simulink model "LADRC2"  (R2023a)
settings: Solver=VariableStepAuto  StartTime=0.0  StopTime=10  RelTol=1e-3
settings Model: Creator=belov  LastModifiedBy=belov

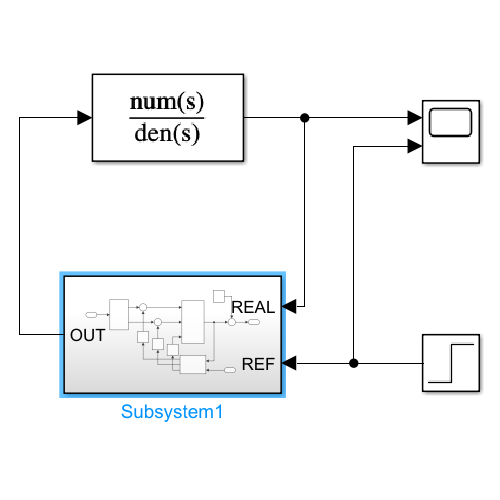
[thumbnail: Simulink's stored preview of the top-level diagram]
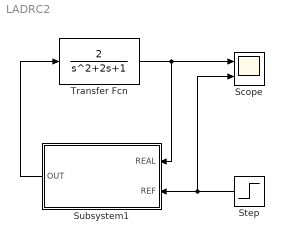
== system LADRC2 ==
  Scope : Scope  NumInputPorts=2
  Step : Step  SampleTime=0.001
  Subsystem1 : Subsystem
  Transfer Fcn : TransferFcn  Numerator=2
  wires:
  Step/1 -> Scope/2, Subsystem1/2(REF)
  Transfer Fcn/1 -> Subsystem1/1(REAL), Scope/1
  Subsystem1/1(OUT) -> Transfer Fcn/1

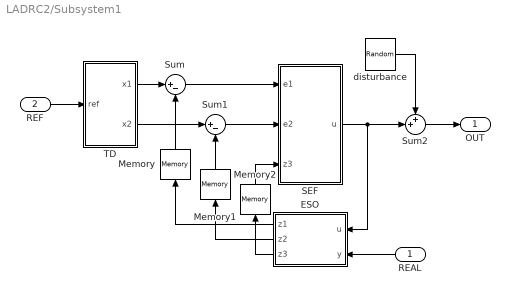
== system LADRC2/Subsystem1 ==
  REAL : Inport
  REF : Inport  Port=2  SampleTime=0.001
  ESO : MATLAB Function  TreatAsAtomicUnit=on  SystemSampleTime=0.001
  Memory : Memory
  Memory1 : Memory
  Memory2 : Memory
  SEF : MATLAB Function  TreatAsAtomicUnit=on  SystemSampleTime=0.001
  Sum : Sum  Inputs=|+-
  Sum1 : Sum  Inputs=|+-
  Sum2 : Sum  Inputs=++|
  TD : MATLAB Function  TreatAsAtomicUnit=on  SystemSampleTime=0.001
  disturbance : UniformRandomNumber  SampleTime=0.1
  OUT : Outport
  wires:
  REAL/1 -> ESO/2(y)
  SEF/1(u) -> Sum2/2, ESO/1(u)
  Sum/1 -> SEF/1(e1)
  Memory1/1 -> Sum1/2
  ESO/2(z2) -> Memory1/1
  Memory/1 -> Sum/2
  TD/1(x1) -> Sum/1
  REF/1 -> TD/1(ref)
  ESO/1(z1) -> Memory/1
  TD/2(x2) -> Sum1/1
  Sum1/1 -> SEF/2(e2)
  ESO/3(z3) -> Memory2/1
  Memory2/1 -> SEF/3(z3)
  disturbance/1 -> Sum2/1
  Sum2/1 -> OUT/1

== matlab function LADRC2/Subsystem1/SEF ==
  data: e1 input; u output; e2 input; z3 input
function u = SEF(e1, e2, z3)

b0 = 1;

wc = 50;

a1 = wc * wc;
a2 = 2 * wc;

u0 = a1 * e1 + a2 * e2;
u = (u0 - z3) / b0;
% u = 1 / b0 * (a1 * e1 + a2 * e2 + a3 * e3 + z4);

end

== matlab function LADRC2/Subsystem1/TD ==
  data: ref input; x1 output; x2 output
function [x1, x2] = TD(ref)

persistent x1_ x2_;

h = 0.001; % 步长
r = 10;

if isempty(x1_)
    x1_=0;
end
if isempty(x2_)
    x2_=0;
end


x1 = x1_ + h * x2_;
x2 = x2_ + h * (-r * r * x1_ - 2 * r * x2_ + r * r * ref);

x1_ = x1;
x2_ = x2;

end

== matlab function LADRC2/Subsystem1/ESO ==
  data: u input; z1 output; y input; z2 output; z3 output
function [z1, z2, z3] = ESO(u, y)

wo = 250;
b0 = 1;

beta1 = 3 * wo;
beta2 = 3 * wo * wo;
beta3 = wo * wo * wo;

h = 0.001;

persistent z1_ z2_ z3_;

if isempty(z1_)
    z1_ = 0;
end
if isempty(z2_)
    z2_ = 0;
end
if isempty(z3_)
    z3_ = 0;
end


z1 = z1_ + h * (-beta1 * z1_ + z2_ + beta1 * y);
z2 = z2_ + h * (-beta2 * z1_ + z3_ + b0 * u + beta2 * y);
z3 = z3_ + h * (-beta3 * z1_ + beta3 * y);

z1_ = z1;
z2_ = z2;
z3_ = z3;
end
